simulink model "simulink_18pulse_diode"  (R2025b)
settings: Solver=FixedStepAuto  StartTime=0.0  StopTime=1.0  RelTol=1e-3
undefined symbols (not defined in the file): plecs
settings Model: Creator=ASUS  LastModifiedBy=ASUS
settings DataIOCC: Refine=5

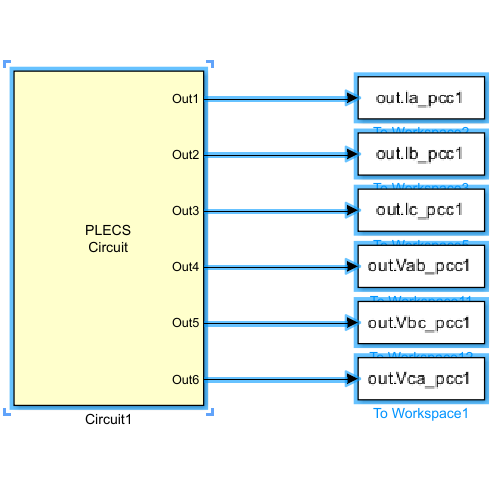
[thumbnail: Simulink's stored preview of the top-level diagram]
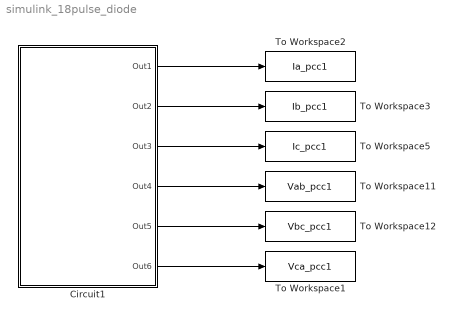
== system simulink_18pulse_diode ==
  Circuit1 : Subsystem  LoadFcn=plecs('sl', 200);  InitFcn=plecs('sl', 214);  StartFcn=plecs('sl', 208);  StopFcn=plecs('sl', 209);  mask(PlecsCircuit){PLECSData=<binary blob, 6036 chars, not shown>}
      mask prompts: PLECSData "PLECS Data (Do not delete or modify!)"
      mask init:
      | % PLACE CUSTOM INITIALIZATIONS ABOVE
      | % DO NOT REMOVE
      | plecs('sl', 215);
      | % DO NOT REMOVE
      settings: CopyFcn=plecs('sl', 203);  DeleteFcn=plecs('sl', 205);  UndoDeleteFcn=plecs('sl', 206);  PreSaveFcn=plecs('sl', 211);  PostSaveFcn=plecs('sl', 201);  NameChangeFcn=plecs('sl', 210);  DestroyFcn=plecs('sl', 207);  PreCopyFcn=plecs('sl', 216);  OpenFcn=plecs('sl', 202);  ErrorFcn=plerrorfcn
      mask Help: eval('plecs(''help'', ''qthelp:///creatingacircuit.html'')')
      mask Display: disp('PLECS\nCircuit')
  To Workspace1 : ToWorkspace  VariableName=Vca_pcc1  SaveFormat=Structure With Time  SampleTime=-1
  To Workspace11 : ToWorkspace  VariableName=Vab_pcc1  SaveFormat=Structure With Time  SampleTime=-1
  To Workspace12 : ToWorkspace  VariableName=Vbc_pcc1  SaveFormat=Structure With Time  SampleTime=-1
  To Workspace2 : ToWorkspace  VariableName=Ia_pcc1  SaveFormat=Structure With Time  SampleTime=-1
  To Workspace3 : ToWorkspace  VariableName=Ib_pcc1  SaveFormat=Structure With Time  SampleTime=-1
  To Workspace5 : ToWorkspace  VariableName=Ic_pcc1  SaveFormat=Structure With Time  SampleTime=-1
  wires:
  Circuit1/1(Out1) -> To Workspace2/1
  Circuit1/2(Out2) -> To Workspace3/1
  Circuit1/3(Out3) -> To Workspace5/1
  Circuit1/4(Out4) -> To Workspace11/1
  Circuit1/5(Out5) -> To Workspace12/1
  Circuit1/6(Out6) -> To Workspace1/1

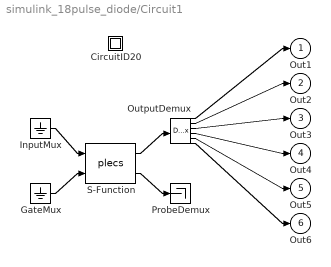
== system simulink_18pulse_diode/Circuit1 ==
  " CircuitID20 " : Subsystem
  " GateMux " : Ground
  " InputMux " : Ground
  " OutputDemux " : Demux  Outputs=[ 1 1 1 1 1 1 ]
  " ProbeDemux " : Terminator
  " S-Function " : S-Function  FunctionName=plecs  SFunctionDeploymentMode=off  EnableBusSupport=off
  Out1 : Outport  PortDimensions=1
  Out2 : Outport  Port=2  PortDimensions=1
  Out3 : Outport  Port=3  PortDimensions=1
  Out4 : Outport  Port=4  PortDimensions=1
  Out5 : Outport  Port=5  PortDimensions=1
  Out6 : Outport  Port=6  PortDimensions=1
  wires:
  " InputMux "/1 -> " S-Function "/1
  " GateMux "/1 -> " S-Function "/2
  " S-Function "/1 -> " OutputDemux "/1
  " S-Function "/2 -> " ProbeDemux "/1
  " OutputDemux "/1 -> Out1/1
  " OutputDemux "/2 -> Out2/1
  " OutputDemux "/3 -> Out3/1
  " OutputDemux "/4 -> Out4/1
  " OutputDemux "/5 -> Out5/1
  " OutputDemux "/6 -> Out6/1

== system simulink_18pulse_diode/Circuit1/ CircuitID20  ==
